simulink subsystem "converter1_filter_r2024a"  (R2024a)
settings: Solver=VariableStepAuto  StartTime=0.0  StopTime=10.0  RelTol=1e-3
libraries: fl_lib x9, nesl_utility x3
settings Model: Creator=chidan  LastModifiedBy=chidan

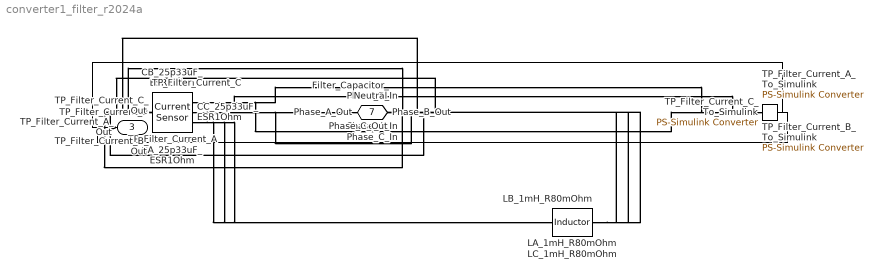
== system converter1_filter_r2024a ==
  CA_25p33uF_ESR1Ohm : fl_lib/Electrical/Electrical Elements/Capacitor  c=25.33029591e-6 F  r=1.0 Ohm  g=0 1/Ohm  i_specify=off  i_priority=None  i=0 A  i_nominal_specify=off  i_nominal_value=1  i_nominal_unit=A  v_specify=off  v_priority=None  v=0 V  v_nominal_specify=off  v_nominal_value=1  v_nominal_unit=V  vc_specify=off  vc_priority=High  vc=0 V  vc_nominal_specify=off  vc_nominal_value=1  vc_nominal_unit=V
  CB_25p33uF_ESR1Ohm : fl_lib/Electrical/Electrical Elements/Capacitor  c=25.33029591e-6 F  r=1.0 Ohm  g=0 1/Ohm  i_specify=off  i_priority=None  i=0 A  i_nominal_specify=off  i_nominal_value=1  i_nominal_unit=A  v_specify=off  v_priority=None  v=0 V  v_nominal_specify=off  v_nominal_value=1  v_nominal_unit=V  vc_specify=off  vc_priority=High  vc=0 V  vc_nominal_specify=off  vc_nominal_value=1  vc_nominal_unit=V
  CC_25p33uF_ESR1Ohm : fl_lib/Electrical/Electrical Elements/Capacitor  c=25.33029591e-6 F  r=1.0 Ohm  g=0 1/Ohm  i_specify=off  i_priority=None  i=0 A  i_nominal_specify=off  i_nominal_value=1  i_nominal_unit=A  v_specify=off  v_priority=None  v=0 V  v_nominal_specify=off  v_nominal_value=1  v_nominal_unit=V  vc_specify=off  vc_priority=High  vc=0 V  vc_nominal_specify=off  vc_nominal_value=1  vc_nominal_unit=V
  LA_1mH_R80mOhm : fl_lib/Electrical/Electrical Elements/Inductor  l=1e-3 H  r=0.08 Ohm  g=1e-9 1/Ohm  i_specify=off  i_priority=None  i=0 A  i_nominal_specify=off  i_nominal_value=1  i_nominal_unit=A  v_specify=off  v_priority=None  v=0 V  v_nominal_specify=off  v_nominal_value=1  v_nominal_unit=V  i_L_specify=off  i_L_priority=High  i_L=0 A  i_L_nominal_specify=off  i_L_nominal_value=1  i_L_nominal_unit=A
  LB_1mH_R80mOhm : fl_lib/Electrical/Electrical Elements/Inductor  l=1e-3 H  r=0.08 Ohm  g=1e-9 1/Ohm  i_specify=off  i_priority=None  i=0 A  i_nominal_specify=off  i_nominal_value=1  i_nominal_unit=A  v_specify=off  v_priority=None  v=0 V  v_nominal_specify=off  v_nominal_value=1  v_nominal_unit=V  i_L_specify=off  i_L_priority=High  i_L=0 A  i_L_nominal_specify=off  i_L_nominal_value=1  i_L_nominal_unit=A
  LC_1mH_R80mOhm : fl_lib/Electrical/Electrical Elements/Inductor  l=1e-3 H  r=0.08 Ohm  g=1e-9 1/Ohm  i_specify=off  i_priority=None  i=0 A  i_nominal_specify=off  i_nominal_value=1  i_nominal_unit=A  v_specify=off  v_priority=None  v=0 V  v_nominal_specify=off  v_nominal_value=1  v_nominal_unit=V  i_L_specify=off  i_L_priority=High  i_L=0 A  i_L_nominal_specify=off  i_L_nominal_value=1  i_L_nominal_unit=A
  TP_Filter_Current_A : fl_lib/Electrical/Electrical Sensors/Current Sensor
  TP_Filter_Current_A_To_Simulink : nesl_utility/PS-Simulink Converter  PhysicalDomain=network_engine_domain  SubClassName=ps_output  LeftPortType=input  RightPortType=output  PseudoPeriodic=off  Frequencies=[]  VectorFormat=inherit  Unit=inherit  AffineConversion=off
  TP_Filter_Current_B : fl_lib/Electrical/Electrical Sensors/Current Sensor
  TP_Filter_Current_B_To_Simulink : nesl_utility/PS-Simulink Converter  PhysicalDomain=network_engine_domain  SubClassName=ps_output  LeftPortType=input  RightPortType=output  PseudoPeriodic=off  Frequencies=[]  VectorFormat=inherit  Unit=inherit  AffineConversion=off
  TP_Filter_Current_C : fl_lib/Electrical/Electrical Sensors/Current Sensor
  TP_Filter_Current_C_To_Simulink : nesl_utility/PS-Simulink Converter  PhysicalDomain=network_engine_domain  SubClassName=ps_output  LeftPortType=input  RightPortType=output  PseudoPeriodic=off  Frequencies=[]  VectorFormat=inherit  Unit=inherit  AffineConversion=off
  Phase_A_In : PMIOPort  Side=Left
  Phase_B_In : PMIOPort  Port=2  Side=Left
  Phase_C_In : PMIOPort  Port=3  Side=Left
  Phase_A_Out : PMIOPort  Port=4  Side=Right
  Phase_B_Out : PMIOPort  Port=5  Side=Right
  Phase_C_Out : PMIOPort  Port=6  Side=Right
  Filter_Capacitor_Neutral : PMIOPort  Port=7  Side=Right
  TP_Filter_Current_A_Out : Outport
  TP_Filter_Current_B_Out : Outport  Port=2
  TP_Filter_Current_C_Out : Outport  Port=3
  wires:
  TP_Filter_Current_A_To_Simulink/1 -> TP_Filter_Current_A_Out/1
  TP_Filter_Current_B_To_Simulink/1 -> TP_Filter_Current_B_Out/1
  TP_Filter_Current_C_To_Simulink/1 -> TP_Filter_Current_C_Out/1
  connections:
  Phase_A_Out/RConn1 -- CA_25p33uF_ESR1Ohm/LConn1 -- LA_1mH_R80mOhm/RConn1
  CA_25p33uF_ESR1Ohm/RConn1 -- CC_25p33uF_ESR1Ohm/RConn1 -- Filter_Capacitor_Neutral/RConn1 -- CB_25p33uF_ESR1Ohm/RConn1
  Phase_B_Out/RConn1 -- CB_25p33uF_ESR1Ohm/LConn1 -- LB_1mH_R80mOhm/RConn1
  Phase_C_Out/RConn1 -- CC_25p33uF_ESR1Ohm/LConn1 -- LC_1mH_R80mOhm/RConn1
  TP_Filter_Current_A/RConn2 -- LA_1mH_R80mOhm/LConn1
  TP_Filter_Current_A/RConn1 -- TP_Filter_Current_A_To_Simulink/LConn1
  TP_Filter_Current_B/RConn2 -- LB_1mH_R80mOhm/LConn1
  TP_Filter_Current_B/RConn1 -- TP_Filter_Current_B_To_Simulink/LConn1
  TP_Filter_Current_C/RConn2 -- LC_1mH_R80mOhm/LConn1
  TP_Filter_Current_C/RConn1 -- TP_Filter_Current_C_To_Simulink/LConn1
  Phase_A_In/RConn1 -- TP_Filter_Current_A/LConn1
  Phase_B_In/RConn1 -- TP_Filter_Current_B/LConn1
  Phase_C_In/RConn1 -- TP_Filter_Current_C/LConn1
